simulink model "cw1sim"  (R2020a)
settings: Solver=VariableStepAuto  StartTime=0.0  StopTime=10.0  RelTol=1e-3
values from neighbouring files (symbols this model uses):
  a = 2    [cw1.m]    (also in model_s.m)
  b = 1    [cw1.m]    (also in model_s.m)
settings Model: Creator=Jan Bronicki  LastModifiedBy=Jan Bronicki

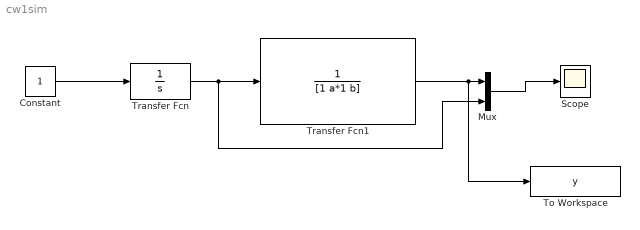
== system cw1sim ==
  Constant : Constant
  Mux : Mux  Inputs=2
  Scope : Scope
  To Workspace : ToWorkspace  VariableName=y  SaveFormat=Timeseries  SampleTime=-1
  Transfer Fcn : TransferFcn  Denominator=[1 0]
  Transfer Fcn1 : TransferFcn  Denominator=[1 a*1 b]
  wires:
  Mux/1 -> Scope/1
  Transfer Fcn1/1 -> To Workspace/1, Mux/1
  Transfer Fcn/1 -> Mux/2, Transfer Fcn1/1
  Constant/1 -> Transfer Fcn/1
